simulink model "cx06_MA"  (Simulink 7.5)
settings: Solver=FixedStepDiscrete  StartTime=0.0  StopTime=10.0  RelTol=1e-3
undefined symbols (not defined in the file or in its folder): DiscIntNeverNeededParam, ECU555, int, motohawk_build_version, motohawk_trunc_name, motohawk_vardec_path
libraries: MotoHawk_lib x811, simulink x43, simulink_need_slupdate x1
(part 6 of 10)

== system cx06_MA/Inputs/Analog Inputs/Trans Inputs ==
  Bus Creator : BusCreator  Inputs=2
  Logical Operator : Logic  Operator=XOR  AllPortsSameDT=off  OutDataTypeMode=boolean  OutDataTypeStr=boolean
  Logical Operator1 : Logic  Operator=XOR  AllPortsSameDT=off  OutDataTypeMode=boolean  OutDataTypeStr=boolean
  motohawk_calibration : MotoHawk_lib/Calibration & Probing Blocks/motohawk_calibration  nam='Neutral_Invert'  val=1  storage=Calibration  show_more=on  name_source=Use Parameter  data_type=Inherit via back propagation  read_level=1  write_level=1  ovr_cals=on  view_as=Enumeration  enum_struct={'False', 'True'}  vector_style=Wide Row  use_help_units=off  help=''  units=''  use_header_enum=off  row_header_enum={}  col_header_enum={}  use_min_max=off  min_val=-inf  max_val=inf  use_precision=off  precision=''  gain=1  offset=0  exp=1  use_mototune_group=off  mototune_group=motohawk_vardec_path(gcb)
  motohawk_calibration1 : MotoHawk_lib/Calibration & Probing Blocks/motohawk_calibration  nam='Reverse_Invert'  val=0  storage=Calibration  show_more=on  name_source=Use Parameter  data_type=Inherit via back propagation  read_level=1  write_level=1  ovr_cals=on  view_as=Enumeration  enum_struct={'False', 'True'}  vector_style=Wide Row  use_help_units=off  help=''  units=''  use_header_enum=off  row_header_enum={}  col_header_enum={}  use_min_max=off  min_val=-inf  max_val=inf  use_precision=off  precision=''  gain=1  offset=0  exp=1  use_mototune_group=off  mototune_group=motohawk_vardec_path(gcb)
  motohawk_din : MotoHawk_lib/Digital I//O Blocks/motohawk_din  resource_name=[]  text_resource=DG1M  code_resource=RES_AN1M  val_resource=-1  target=ECU555-80  resource_enum_str=(None)=-1,AN1M=56,AN2M=57,AN3M=58,AN4M=59,AN5M=60,AN6M=61,AN7M=62,AN8M=63,AN9M=64,AN10M=65,AN11M=66,AN12M=67,AN13M=68,AN14M=69,AN15M=70,AN16M=71,AN17M=72,AN18M=73,AN19M=74,O2A=90,O2B=91,DG1M=93,DG2M=94,DG4M=96,ESTOP=97  pullup=None  use_stat=on  use_vardec=on  nam='Neutral'  read_level=1  write_level=1  group='I/O Pins | Inputs Config'
  motohawk_din1 : MotoHawk_lib/Digital I//O Blocks/motohawk_din  resource_name=[]  text_resource=AN3M  code_resource=RES_AN1M  val_resource=-1  target=ECU555-80  resource_enum_str=(None)=-1,AN1M=56,AN2M=57,AN3M=58,AN4M=59,AN5M=60,AN6M=61,AN7M=62,AN8M=63,AN9M=64,AN10M=65,AN11M=66,AN12M=67,AN13M=68,AN14M=69,AN15M=70,AN16M=71,AN17M=72,AN18M=73,AN19M=74,O2A=90,O2B=91,DG1M=93,DG2M=94,DG4M=96,ESTOP=97  pullup=None  use_stat=on  use_vardec=on  nam='Reverse'  read_level=1  write_level=1  group='I/O Pins | Inputs Config'
  motohawk_probe : MotoHawk_lib/Calibration & Probing Blocks/motohawk_probe  nam='cal_Neutral'  show_more=on  name_source=Use Parameter  read_level=1  view_as=Enumeration  enum_struct={'False', 'True'}  vector_style=Wide Row  use_help_units=off  help=''  units=''  use_header_enum=off  row_header_enum={}  col_header_enum={}  use_precision=off  precision=''  gain=1  offset=0  exp=1  use_mototune_group=off  mototune_group=motohawk_vardec_path(gcb)
  motohawk_probe1 : MotoHawk_lib/Calibration & Probing Blocks/motohawk_probe  nam='cal_Reverse'  show_more=on  name_source=Use Parameter  read_level=1  view_as=Enumeration  enum_struct={'False', 'True'}  vector_style=Wide Row  use_help_units=off  help=''  units=''  use_header_enum=off  row_header_enum={}  col_header_enum={}  use_precision=off  precision=''  gain=1  offset=0  exp=1  use_mototune_group=off  mototune_group=motohawk_vardec_path(gcb)
  motohawk_probe2 : MotoHawk_lib/Calibration & Probing Blocks/motohawk_probe  nam='Err_Reverse'  show_more=on  name_source=Use Parameter  read_level=1  view_as=Number  enum_struct={'Disabled', 'Enabled'}  vector_style=Wide Row  use_help_units=off  help=''  units=''  use_header_enum=off  row_header_enum={}  col_header_enum={}  use_precision=off  precision=''  gain=1  offset=0  exp=1  use_mototune_group=on  mototune_group='Debug | Inputs'
  motohawk_probe3 : MotoHawk_lib/Calibration & Probing Blocks/motohawk_probe  nam='Err_Neutral'  show_more=on  name_source=Use Parameter  read_level=1  view_as=Number  enum_struct={'Disabled', 'Enabled'}  vector_style=Wide Row  use_help_units=off  help=''  units=''  use_header_enum=off  row_header_enum={}  col_header_enum={}  use_precision=off  precision=''  gain=1  offset=0  exp=1  use_mototune_group=on  mototune_group='Debug | Inputs'
  Trans : Outport  OutDataType=sfix(16)  OutScaling=2^0
  wires:
  Bus Creator/1 -> Trans/1
  motohawk_calibration/1 -> Logical Operator/1
  motohawk_din/1 -> Logical Operator/2
  Logical Operator/1 -> Bus Creator/1, motohawk_probe/1  "Neutral"
  motohawk_calibration1/1 -> Logical Operator1/1
  motohawk_din1/1 -> Logical Operator1/2
  Logical Operator1/1 -> motohawk_probe1/1, Bus Creator/2  "Reverse"
  motohawk_din/2 -> motohawk_probe3/1
  motohawk_din1/2 -> motohawk_probe2/1

== system cx06_MA/Inputs/GMLAN Inputs/Valid_Chk ==
  In : Inport  OutDataType=sfix(16)  OutScaling=2^0
  Valid : Inport  Port=2  OutDataType=sfix(16)  OutScaling=2^0
  Switch : Switch  Criteria=u2 ~= 0
  Unit Delay : UnitDelay  SampleTime=-1
  Out1 : Outport  OutDataType=sfix(16)  OutScaling=2^0
  wires:
  Valid/1 -> Switch/2
  In/1 -> Switch/3
  Unit Delay/1 -> Switch/1
  Switch/1 -> Unit Delay/1, Out1/1

== system cx06_MA/Inputs/GMLAN Inputs/Valid_Chk1 ==
  In : Inport  OutDataType=sfix(16)  OutScaling=2^0
  Valid : Inport  Port=2  OutDataType=sfix(16)  OutScaling=2^0
  Switch : Switch  Criteria=u2 ~= 0
  Unit Delay : UnitDelay  SampleTime=-1
  Out1 : Outport  OutDataType=sfix(16)  OutScaling=2^0
  wires:
  Switch/1 -> Out1/1, Unit Delay/1
  Unit Delay/1 -> Switch/1
  In/1 -> Switch/3
  Valid/1 -> Switch/2

== system cx06_MA/Inputs/GMLAN Inputs/Valid_Chk2 ==
  In : Inport  OutDataType=sfix(16)  OutScaling=2^0
  Valid : Inport  Port=2  OutDataType=sfix(16)  OutScaling=2^0
  Switch : Switch  Criteria=u2 ~= 0
  Unit Delay : UnitDelay  SampleTime=-1
  Out1 : Outport  OutDataType=sfix(16)  OutScaling=2^0
  wires:
  Valid/1 -> Switch/2
  In/1 -> Switch/3
  Unit Delay/1 -> Switch/1
  Switch/1 -> Unit Delay/1, Out1/1

== system cx06_MA/Inputs/GMLAN Inputs/Valid_Chk3 ==
  In : Inport  OutDataType=sfix(16)  OutScaling=2^0
  Valid : Inport  Port=2  OutDataType=sfix(16)  OutScaling=2^0
  Switch : Switch  Criteria=u2 ~= 0
  Unit Delay : UnitDelay  SampleTime=-1
  Out1 : Outport  OutDataType=sfix(16)  OutScaling=2^0
  wires:
  Switch/1 -> Out1/1, Unit Delay/1
  Unit Delay/1 -> Switch/1
  In/1 -> Switch/3
  Valid/1 -> Switch/2

== system cx06_MA/Inputs/IPT CAN Input/speed_calc ==
  whl_rpm : Inport  OutDataType=sfix(16)  OutScaling=2^0
  gear_ratio : Inport  Port=2  OutDataType=sfix(16)  OutScaling=2^0
  Constant : Constant  Value=pi()/12/5280*60  OutDataType=sfix(16)  OutScaling=2^0
  Divide : Product  Inputs=***/  OutDataType=sfix(16)  OutScaling=2^-10
  motohawk_calibration : MotoHawk_lib/Calibration & Probing Blocks/motohawk_calibration  nam='Tire_Size'  val=26  storage=Calibration  show_more=on  name_source=Use Parameter  data_type=Inherit from 'Default Value'  read_level=1  write_level=1  ovr_cals=on  view_as=Number  enum_struct={'Disabled', 'Enabled'}  vector_style=Wide Row  use_help_units=on  help='Tire Diameter (used to calculate vehicle speed'  units='in'  use_header_enum=off  row_header_enum={}  col_header_enum={}  use_min_max=off  min_val=0  max_val=100  use_precision=on  precision='2.2'  gain=1  offset=0  exp=1  use_mototune_group=off  mototune_group=motohawk_vardec_path(gcb)
  Veh_mph : Outport  OutDataType=sfix(16)  OutScaling=2^0
  wires:
  whl_rpm/1 -> Divide/1
  Constant/1 -> Divide/2
  motohawk_calibration/1 -> Divide/3
  Divide/1 -> Veh_mph/1
  gear_ratio/1 -> Divide/4

== system cx06_MA/Outputs/Analog Outputs/Backup_Relay_Control ==
  Engine_Start_In : Inport  OutDataType=sfix(16)  OutScaling=2^0
  Chart : Stateflow chart  TreatAsAtomicUnit=on
  Data Type Conversion : DataTypeConversion  OutDataTypeMode=boolean  OutDataType=sfix(16)  OutScaling=2^0  OutDataTypeStr=boolean
  Data Type Conversion1 : DataTypeConversion  OutDataTypeMode=boolean  OutDataType=sfix(16)  OutScaling=2^0  OutDataTypeStr=boolean
  Subsystem : Subsystem
  Unit Delay : UnitDelay  SampleTime=-1
  motohawk_calibration : MotoHawk_lib/Calibration & Probing Blocks/motohawk_calibration  nam='Idle_to_Crank_Delay'  val=5  storage=Calibration  show_more=on  name_source=Use Parameter  data_type=uint16  read_level=1  write_level=1  ovr_cals=on  view_as=Number  enum_struct={'Disabled', 'Enabled'}  vector_style=Wide Row  use_help_units=on  help=''  units='ms'  use_header_enum=off  row_header_enum={}  col_header_enum={}  use_min_max=on  min_val=0  max_val=1000  use_precision=on  precision=''  gain=1/5  offset=0  exp=1  use_mototune_group=off  mototune_group=motohawk_vardec_path(gcb)
  motohawk_calibration1 : MotoHawk_lib/Calibration & Probing Blocks/motohawk_calibration  nam='Crank_to_Idle_Delay'  val=5  storage=Calibration  show_more=on  name_source=Use Parameter  data_type=uint16  read_level=1  write_level=1  ovr_cals=on  view_as=Number  enum_struct={'Disabled', 'Enabled'}  vector_style=Wide Row  use_help_units=on  help=''  units='ms'  use_header_enum=off  row_header_enum={}  col_header_enum={}  use_min_max=on  min_val=0  max_val=1000  use_precision=on  precision=''  gain=1/5  offset=0  exp=1  use_mototune_group=off  mototune_group=motohawk_vardec_path(gcb)
  motohawk_probe : MotoHawk_lib/Calibration & Probing Blocks/motohawk_probe  nam='KevOBox_State'  show_more=on  name_source=Use Parameter  read_level=1  view_as=Enumeration  enum_struct={'Idle', 'About_to_Crank', 'Crank', 'About_to_Idle'}  vector_style=Wide Row  use_help_units=off  help=''  units=''  use_header_enum=off  row_header_enum={}  col_header_enum={}  use_precision=off  precision=''  gain=1  offset=0  exp=1  use_mototune_group=off  mototune_group=motohawk_vardec_path(gcb)
  motohawk_probe1 : MotoHawk_lib/Calibration & Probing Blocks/motohawk_probe  nam='Timer'  show_more=on  name_source=Use Parameter  read_level=1  view_as=Number  enum_struct={'Idle', 'About_to_Crank',Crank',About_to_Idle'}  vector_style=Wide Row  use_help_units=off  help=''  units=''  use_header_enum=off  row_header_enum={}  col_header_enum={}  use_precision=off  precision=''  gain=1  offset=0  exp=1  use_mototune_group=off  mototune_group=motohawk_vardec_path(gcb)
  Engine_Start_Out : Outport  OutDataType=sfix(16)  OutScaling=2^0
  Clarion_Pwr_Out : Outport  Port=2  OutDataType=sfix(16)  OutScaling=2^0
  wires:
  motohawk_calibration/1 -> Subsystem/2(Idle_to_Crank Cal)
  motohawk_calibration1/1 -> Subsystem/3(Crank_to_Idle Cal)
  Chart/4(state) -> motohawk_probe/1
  Chart/3(timer) -> Unit Delay/1
  Chart/1(LSD_Eng) -> Data Type Conversion/1
  Chart/2(LSD_Nav) -> Data Type Conversion1/1
  Subsystem/2(Idle_to_Crank Delay) -> Chart/2(Delay_1)
  Subsystem/3(Crank_to_Idle Delay) -> Chart/3(Delay_2)
  Subsystem/1(Timer) -> motohawk_probe1/1
  Engine_Start_In/1 -> Chart/1(Eng_Start)
  Data Type Conversion1/1 -> Clarion_Pwr_Out/1
  Data Type Conversion/1 -> Engine_Start_Out/1
  Unit Delay/1 -> Subsystem/1(timer_en)

== system cx06_MA/Outputs/Analog Outputs/Nav Sys Timer ==
  Constant1 : Constant  OutDataType=sfix(16)  OutScaling=2^0
  Gain1 : Gain  Gain=1/200  ParameterDataType=sfix(16)  ParameterScaling=2^0  OutDataType=sfix(16)  OutScaling=2^0
  Relational Operator1 : RelationalOperator  Operator=>  LogicOutDataTypeMode=Specify via dialog  OutDataTypeStr=uint(8)
  Saturation : Saturate  UpperLimit=6000  LowerLimit=0
  Sum : Sum  Inputs=|++  OutDataType=sfix(16)  OutScaling=2^0
  Unit Delay : UnitDelay  X0=1  SampleTime=-1
  motohawk_calibration2 : MotoHawk_lib/Calibration & Probing Blocks/motohawk_calibration  nam='Disable_Nav_Safety_Delay'  val=3000  storage=Calibration  show_more=on  name_source=Use Parameter  data_type=double  read_level=1  write_level=1  ovr_cals=on  view_as=Number  enum_struct={'False', 'True'}  vector_style=Wide Row  use_help_units=on  help='time which requested IPT Torque has to be below Zero_Threshold before disabling MCU'  units='sec'  use_header_enum=off  row_header_enum={}  col_header_enum={}  use_min_max=on  min_val=0  max_val=6000  use_precision=on  precision='1.3'  gain=1/200  offset=0  exp=1  use_mototune_group=off  mototune_group=motohawk_vardec_path(gcb)
  motohawk_probe1 : MotoHawk_lib/Calibration & Probing Blocks/motohawk_probe  nam='Nav_Cnt_Seconds'  show_more=off  name_source=Use Parameter  read_level=1  view_as=Number  enum_struct={'Disabled', 'Enabled'}  vector_style=Wide Row  use_help_units=off  help=''  units=''  use_header_enum=off  row_header_enum={}  col_header_enum={}  use_precision=off  precision=''  gain=1  offset=0  exp=1  use_mototune_group=off  mototune_group=motohawk_vardec_path(gcb)
  Out : Outport  OutDataType=sfix(16)  OutScaling=2^0
  wires:
  motohawk_calibration2/1 -> Relational Operator1/2
  Relational Operator1/1 -> Out/1
  Sum/1 -> Saturation/1
  Saturation/1 -> Unit Delay/1, Relational Operator1/1, Gain1/1
  Unit Delay/1 -> Sum/1
  Constant1/1 -> Sum/2
  Gain1/1 -> motohawk_probe1/1

== system cx06_MA/Outputs/Drive-by-Wire CAN Output/Subsystem ==
  Reset_AO1 : Inport  OutDataType=sfix(16)  OutScaling=2^0
  Output1 : Inport  Port=2  OutDataType=sfix(16)  OutScaling=2^0
  Reset_AO2 : Inport  Port=3  OutDataType=sfix(16)  OutScaling=2^0
  Output2 : Inport  Port=4  OutDataType=sfix(16)  OutScaling=2^0
  Bitwise Operator : simulink/Logic and Bit Operations/Bitwise Operator  logicop=AND  UseBitMask=on  BitMask=1  BitMaskRealWorld=Stored Integer
  Bitwise Operator1 : simulink/Logic and Bit Operations/Bitwise Operator  logicop=AND  UseBitMask=on  BitMask=1  BitMaskRealWorld=Stored Integer
  Bitwise Operator2 : simulink/Logic and Bit Operations/Bitwise Operator  logicop=AND  UseBitMask=on  BitMask=hex2dec('FFF')  BitMaskRealWorld=Stored Integer
  Bitwise Operator3 : simulink/Logic and Bit Operations/Bitwise Operator  logicop=OR  UseBitMask=off  NumInputPorts=2  BitMask=hex2dec('FFF')  BitMaskRealWorld=Stored Integer
  Bitwise Operator4 : simulink/Logic and Bit Operations/Bitwise Operator  logicop=AND  UseBitMask=on  BitMask=hex2dec('FFF')  BitMaskRealWorld=Stored Integer
  Bitwise Operator5 : simulink/Logic and Bit Operations/Bitwise Operator  logicop=OR  UseBitMask=off  NumInputPorts=2  BitMask=hex2dec('FFF')  BitMaskRealWorld=Stored Integer
  Bitwise Operator6 : simulink/Logic and Bit Operations/Bitwise Operator  logicop=XOR  UseBitMask=off  NumInputPorts=4  BitMask=hex2dec('FFF')  BitMaskRealWorld=Stored Integer
  Extract Bits : simulink/Logic and Bit Operations/Extract Bits  SystemSampleTime=-1  bitsToExtract=Range starting with most significant bit  numBits=8  bitIdxRange=[0 7]  outScalingMode=Treat bit field as an integer
  Extract Bits1 : simulink/Logic and Bit Operations/Extract Bits  SystemSampleTime=-1  bitsToExtract=Range ending with least significant bit  numBits=8  bitIdxRange=[0 7]  outScalingMode=Treat bit field as an integer
  Extract Bits2 : simulink/Logic and Bit Operations/Extract Bits  SystemSampleTime=-1  bitsToExtract=Range starting with most significant bit  numBits=8  bitIdxRange=[0 7]  outScalingMode=Treat bit field as an integer
  Extract Bits3 : simulink/Logic and Bit Operations/Extract Bits  SystemSampleTime=-1  bitsToExtract=Range ending with least significant bit  numBits=8  bitIdxRange=[0 7]  outScalingMode=Treat bit field as an integer
  Shift Arithmetic : simulink/Logic and Bit Operations/Shift Arithmetic  SystemSampleTime=-1  nBitShiftRight=-4  nBinPtShiftRight=0
  Checksum : Outport  OutDataType=sfix(16)  OutScaling=2^0
  wires:
  Reset_AO1/1 -> Bitwise Operator/1
  Bitwise Operator/1 -> Shift Arithmetic/1
  Reset_AO2/1 -> Bitwise Operator1/1
  Shift Arithmetic/1 -> Bitwise Operator3/1
  Bitwise Operator2/1 -> Bitwise Operator3/2
  Bitwise Operator4/1 -> Bitwise Operator5/2
  Output2/1 -> Bitwise Operator4/1
  Bitwise Operator1/1 -> Bitwise Operator5/1
  Bitwise Operator3/1 -> Extract Bits/1, Extract Bits1/1
  Bitwise Operator5/1 -> Extract Bits2/1, Extract Bits3/1
  Extract Bits/1 -> Bitwise Operator6/1
  Extract Bits1/1 -> Bitwise Operator6/2
  Extract Bits2/1 -> Bitwise Operator6/3
  Extract Bits3/1 -> Bitwise Operator6/4
  Bitwise Operator6/1 -> Checksum/1
  Output1/1 -> Bitwise Operator2/1

== system cx06_MA/Outputs/GMLAN Outputs/Fuel/SOC_Gage_Conditioning ==
  In1 : Inport  OutDataType=sfix(16)  OutScaling=2^0
  Bus Selector2 : BusSelector  OutputSignals=Analog.Fuel_Level,Analog.cruiseBut,JCI.SOC
  Constant : Constant  Value=0  OutDataType=sfix(16)  OutScaling=2^0
  Constant1 : Constant  OutDataType=fixdt(1, 16)  OutScaling=2^0
  Constant2 : Constant  Value=0  OutDataType=sfix(16)  OutScaling=2^0
  Constant3 : Constant  OutDataType=sfix(16)  OutScaling=2^0
  Fuel_Signal_Conditioning : Subsystem
  Gain : Gain  Gain=100  ParameterDataType=sfix(16)  ParameterScaling=2^0  OutDataType=sfix(16)  OutScaling=2^0
  Logical Operator : Logic  Operator=NOT  AllPortsSameDT=off  OutDataTypeMode=Specify via dialog  OutDataTypeStr=uint(8)
  Mux4 : Mux  Inputs=3
  Relational Operator : RelationalOperator  Operator===  LogicOutDataTypeMode=boolean  OutDataTypeStr=boolean
  Relational Operator1 : RelationalOperator  Operator===  LogicOutDataTypeMode=boolean  OutDataTypeStr=boolean
  Relational Operator2 : RelationalOperator  Operator===  LogicOutDataTypeMode=boolean  OutDataTypeStr=boolean
  Saturation : Saturate  UpperLimit=1000  LowerLimit=0
  Saturation1 : Saturate  UpperLimit=100  LowerLimit=0
  Saturation3 : Saturate  UpperLimit=100  LowerLimit=0
  Sum : Sum  Inputs=-+  OutDataType=sfix(16)  OutScaling=2^0
  Sum1 : Sum  Inputs=|++  OutDataType=sfix(16)  OutScaling=2^0
  Switch{,1..3} (4 alike) : Switch  Threshold=1
  Unit Delay : UnitDelay  X0=1  SampleTime=-1
  Unit Delay1 : UnitDelay  X0=1001  SampleTime=-1
  motohawk_calibration : MotoHawk_lib/Calibration & Probing Blocks/motohawk_calibration  nam='Gage_Delay'  val=0  storage=Calibration  show_more=on  name_source=Use Parameter  data_type=Inherit from 'Default Value'  read_level=1  write_level=1  ovr_cals=on  view_as=Number  enum_struct={'Disabled', 'Enabled'}  vector_style=Wide Row  use_help_units=off  help=''  units=''  use_header_enum=off  row_header_enum={}  col_header_enum={}  use_min_max=on  min_val=0  max_val=5  use_precision=on  precision='1.3'  gain=1/200  offset=0  exp=1  use_mototune_group=off  mototune_group=motohawk_vardec_path(gcb)
  motohawk_calibration1 : MotoHawk_lib/Calibration & Probing Blocks/motohawk_calibration  nam='TransGoToPoint'  val=12  storage=Calibration  show_more=on  name_source=Use Parameter  data_type=Inherit from 'Default Value'  read_level=1  write_level=1  ovr_cals=on  view_as=Number  enum_struct={'Disabled', 'Enabled'}  vector_style=Wide Row  use_help_units=off  help=''  units=''  use_header_enum=off  row_header_enum={}  col_header_enum={}  use_min_max=on  min_val=0  max_val=100  use_precision=on  precision='1.3'  gain=1  offset=0  exp=1  use_mototune_group=off  mototune_group=motohawk_vardec_path(gcb)
  motohawk_calibration2 : MotoHawk_lib/Calibration & Probing Blocks/motohawk_calibration  nam='Bat_Lvl_Offset'  val=0  storage=Calibration  show_more=on  name_source=Use Parameter  data_type=Inherit from 'Default Value'  read_level=1  write_level=1  ovr_cals=on  view_as=Number  enum_struct={'Disabled', 'Enabled'}  vector_style=Wide Row  use_help_units=off  help=''  units=''  use_header_enum=off  row_header_enum={}  col_header_enum={}  use_min_max=on  min_val=0  max_val=100  use_precision=on  precision='1.3'  gain=1  offset=0  exp=1  use_mototune_group=off  mototune_group=motohawk_vardec_path(gcb)
  motohawk_calibration7 : MotoHawk_lib/Calibration & Probing Blocks/motohawk_calibration  nam='SOC_Lvl_Zero'  val=5  storage=Calibration  show_more=on  name_source=Use Parameter  data_type=Inherit via back propagation  read_level=1  write_level=1  ovr_cals=on  view_as=Number  enum_struct={'Disabled', 'Enabled'}  vector_style=Wide Row  use_help_units=off  help=''  units=''  use_header_enum=off  row_header_enum={}  col_header_enum={}  use_min_max=off  min_val=-inf  max_val=inf  use_precision=off  precision=''  gain=1  offset=0  exp=1  use_mototune_group=off  mototune_group=motohawk_vardec_path(gcb)
  motohawk_calibration8 : MotoHawk_lib/Calibration & Probing Blocks/motohawk_calibration  nam='SOC_Lvl_Full'  val=100  storage=Calibration  show_more=on  name_source=Use Parameter  data_type=Inherit via back propagation  read_level=1  write_level=1  ovr_cals=on  view_as=Number  enum_struct={'Disabled', 'Enabled'}  vector_style=Wide Row  use_help_units=off  help=''  units=''  use_header_enum=off  row_header_enum={}  col_header_enum={}  use_min_max=off  min_val=-inf  max_val=inf  use_precision=off  precision=''  gain=1  offset=0  exp=1  use_mototune_group=off  mototune_group=motohawk_vardec_path(gcb)
  motohawk_probe : MotoHawk_lib/Calibration & Probing Blocks/motohawk_probe  nam='Bat_Lvl_Out'  show_more=off  name_source=Use Parameter  read_level=1  view_as=Number  enum_struct={'Disabled', 'Enabled'}  vector_style=Wide Row  use_help_units=off  help=''  units=''  use_header_enum=off  row_header_enum={}  col_header_enum={}  use_precision=off  precision=''  gain=1  offset=0  exp=1  use_mototune_group=off  mototune_group=motohawk_vardec_path(gcb)
  motohawk_probe1 : MotoHawk_lib/Calibration & Probing Blocks/motohawk_probe  nam='Fuel_Lvl_Out'  show_more=off  name_source=Use Parameter  read_level=1  view_as=Number  enum_struct={'Disabled', 'Enabled'}  vector_style=Wide Row  use_help_units=off  help=''  units=''  use_header_enum=off  row_header_enum={}  col_header_enum={}  use_precision=off  precision=''  gain=1  offset=0  exp=1  use_mototune_group=off  mototune_group=motohawk_vardec_path(gcb)
  motohawk_probe2 : MotoHawk_lib/Calibration & Probing Blocks/motohawk_probe  nam='Delay_Count'  show_more=off  name_source=Use Parameter  read_level=1  view_as=Number  enum_struct={'Disabled', 'Enabled'}  vector_style=Wide Row  use_help_units=off  help=''  units=''  use_header_enum=off  row_header_enum={}  col_header_enum={}  use_precision=off  precision=''  gain=1  offset=0  exp=1  use_mototune_group=off  mototune_group=motohawk_vardec_path(gcb)
  my2pt Cal : Fcn  Expr=(u[1]-u[3])/(u[2]-u[3])
  Out1 : Outport  OutDataType=sfix(16)  OutScaling=2^0
  wires:
  In1/1 -> Bus Selector2/1
  Bus Selector2/1 -> Fuel_Signal_Conditioning/1(Fuel_Level)  "<Fuel_Level>"
  Bus Selector2/2 -> Relational Operator/1  "<cruiseBut>"
  Constant/1 -> Relational Operator/2, Switch3/1
  Relational Operator/1 -> Switch/2, Unit Delay/1, Relational Operator1/1
  Fuel_Signal_Conditioning/1(Out1) -> Switch/1, motohawk_probe1/1
  Switch/1 -> Switch1/1
  Unit Delay/1 -> Relational Operator1/2
  Constant2/1 -> Relational Operator2/1
  Relational Operator2/1 -> Switch1/2
  Saturation/1 -> Relational Operator2/2, Unit Delay1/1, motohawk_probe2/1
  Sum/1 -> Saturation/1
  Constant3/1 -> Sum/1
  Relational Operator1/1 -> Switch2/2
  Unit Delay1/1 -> Switch2/1
  motohawk_calibration/1 -> Switch2/3
  Switch2/1 -> Sum/2
  Mux4/1 -> my2pt Cal/1
  motohawk_calibration7/1 -> Mux4/3
  motohawk_calibration8/1 -> Mux4/2
  Bus Selector2/3 -> Mux4/1  "<SOC>"
  motohawk_calibration1/1 -> Switch1/3
  Switch1/1 -> Out1/1
  motohawk_calibration2/1 -> Sum1/2
  Switch3/1 -> Switch/3
  Saturation3/1 -> Switch3/3
  Logical Operator/1 -> Switch3/2
  my2pt Cal/1 -> Gain/1
  Gain/1 -> Saturation1/1
  Sum1/1 -> Saturation3/1, motohawk_probe/1
  Saturation1/1 -> Sum1/1
  Constant1/1 -> Logical Operator/1

== system cx06_MA/Outputs/GMLAN Outputs/Speed_Integrator ==
  In1 : Inport  OutDataType=sfix(16)  OutScaling=2^0
  Compare To Constant : simulink/Logic and Bit Operations/Compare To Constant  SystemSampleTime=-1  relop=>  const=1000  LogicOutDataTypeMode=uint8  ZeroCross=off
  Compare To Constant1 : simulink/Logic and Bit Operations/Compare To Constant  SystemSampleTime=-1  relop=<  const=5  LogicOutDataTypeMode=uint8  ZeroCross=off
  Gain : Gain  Gain=1/(60*60*200)  ParameterDataType=sfix(16)  ParameterScaling=2^0  OutDataType=sfix(16)  OutScaling=2^0
  Logical Operator : Logic  Operator=NOT  AllPortsSameDT=off  OutDataTypeMode=Specify via dialog  OutDataTypeStr=uint(8)
  Logical Operator1 : Logic  Operator=OR  AllPortsSameDT=off  OutDataTypeMode=Specify via dialog  OutDataTypeStr=uint(8)
  Product : Product  OutDataType=sfix(16)  OutScaling=2^0  RndMeth=Zero
  Sum : Sum  Inputs=|++  OutDataType=sfix(16)  OutScaling=2^0
  Unit Delay : UnitDelay  SampleTime=-1
  Reset : Outport  OutDataType=sfix(16)  OutScaling=2^0
  Out1 : Outport  Port=2  OutDataType=sfix(16)  OutScaling=2^0
  wires:
  In1/1 -> Gain/1
  Gain/1 -> Sum/1
  Unit Delay/1 -> Sum/2
  Sum/1 -> Compare To Constant/1, Product/1, Out1/1, Compare To Constant1/1
  Compare To Constant/1 -> Logical Operator/1, Logical Operator1/2
  Product/1 -> Unit Delay/1
  Logical Operator/1 -> Product/2
  Logical Operator1/1 -> Reset/1
  Compare To Constant1/1 -> Logical Operator1/1

== system cx06_MA/Outputs/GMLAN Outputs/Subsystem ==
  Engine_Running : Inport  OutDataType=sfix(16)  OutScaling=2^0
  Constant : Constant  OutDataType=sfix(16)  OutScaling=2^0
  Switch : Switch  Criteria=u2 ~= 0
  motohawk_fault_action : MotoHawk_lib/Fault Management Blocks/motohawk_fault_action  nam='Clutch'  output_status=on  eval_nam=Clutch
  Out1 : Outport  OutDataType=sfix(16)  OutScaling=2^0
  wires:
  motohawk_fault_action/1 -> Switch/2
  Constant/1 -> Switch/3
  Engine_Running/1 -> Switch/1
  Switch/1 -> Out1/1

== system cx06_MA/Outputs/IPT CAN Output/MCU_Management ==
  Motor_Torque_Request : Inport  OutDataType=sfix(16)  OutScaling=2^0
  MCU_Enable_IN : Inport  Port=2  OutDataType=sfix(16)  OutScaling=2^0
  Abs : Abs
  Constant : Constant  Value=0  OutDataType=sfix(16)  OutScaling=2^0
  Constant1 : Constant  OutDataType=sfix(16)  OutScaling=2^0
  Data Type Conversion : DataTypeConversion  OutDataTypeMode=uint8  OutDataType=sfix(16)  OutScaling=2^0  OutDataTypeStr=uint8
  Gain1 : Gain  Gain=1/200  ParameterDataType=sfix(16)  ParameterScaling=2^0  OutDataType=sfix(16)  OutScaling=2^0
  Logical Operator : Logic  Operator=OR  AllPortsSameDT=off  OutDataTypeMode=boolean  OutDataTypeStr=boolean
  Relational Operator : RelationalOperator  Operator=<  LogicOutDataTypeMode=Specify via dialog  OutDataTypeStr=uint(8)
  Relational Operator1 : RelationalOperator  Operator=<  LogicOutDataTypeMode=Specify via dialog  OutDataTypeStr=uint(8)
  Saturation : Saturate  UpperLimit=6000  LowerLimit=0
  Sum : Sum  Inputs=|++  OutDataType=sfix(16)  OutScaling=2^0
  Switch : Switch  Criteria=u2 > Threshold  OutDataTypeStr=Inherit: Inherit via back propagation  RndMeth=Nearest
  Switch1 : Switch  Criteria=u2 > Threshold  OutDataTypeStr=Inherit: Inherit via back propagation
  Unit Delay : UnitDelay  X0=1  SampleTime=-1
  motohawk_calibration1 : MotoHawk_lib/Calibration & Probing Blocks/motohawk_calibration  nam='MCU_Manage_Source'  val=0  storage=Calibration  show_more=on  name_source=Use Parameter  data_type=uint8  read_level=1  write_level=1  ovr_cals=on  view_as=Enumeration  enum_struct={'By_State', 'By_Torque_Dmd'}  vector_style=Wide Row  use_help_units=off  help=''  units=''  use_header_enum=off  row_header_enum={}  col_header_enum={}  use_min_max=on  min_val=0  max_val=1  use_precision=off  precision=''  gain=1  offset=0  exp=1  use_mototune_group=off  mototune_group=motohawk_vardec_path(gcb)
  motohawk_calibration11 : MotoHawk_lib/Calibration & Probing Blocks/motohawk_calibration  nam='Zero_Threshold'  val=.01  storage=Calibration  show_more=on  name_source=Use Parameter  data_type=double  read_level=1  write_level=1  ovr_cals=on  view_as=Number  enum_struct={'False', 'True'}  vector_style=Wide Row  use_help_units=off  help=''  units=''  use_header_enum=off  row_header_enum={}  col_header_enum={}  use_min_max=on  min_val=0  max_val=1  use_precision=on  precision='1.3'  gain=1  offset=0  exp=1  use_mototune_group=off  mototune_group=motohawk_vardec_path(gcb)
  motohawk_calibration2 : MotoHawk_lib/Calibration & Probing Blocks/motohawk_calibration  nam='Disable_MCU_Delay'  val=1200  storage=Calibration  show_more=on  name_source=Use Parameter  data_type=double  read_level=1  write_level=1  ovr_cals=on  view_as=Number  enum_struct={'False', 'True'}  vector_style=Wide Row  use_help_units=on  help='time which requested IPT Torque has to be below Zero_Threshold before disabling MCU'  units='sec'  use_header_enum=off  row_header_enum={}  col_header_enum={}  use_min_max=on  min_val=0  max_val=6000  use_precision=on  precision='1.3'  gain=1/200  offset=0  exp=1  use_mototune_group=off  mototune_group=motohawk_vardec_path(gcb)
  motohawk_calibration3 : MotoHawk_lib/Calibration & Probing Blocks/motohawk_calibration  nam='Inhibit_MCU_Management'  val=1  storage=Calibration  show_more=on  name_source=Use Parameter  data_type=uint8  read_level=1  write_level=1  ovr_cals=on  view_as=Enumeration  enum_struct={'False', 'True'}  vector_style=Wide Row  use_help_units=off  help=''  units=''  use_header_enum=off  row_header_enum={}  col_header_enum={}  use_min_max=on  min_val=0  max_val=1  use_precision=off  precision=''  gain=1  offset=0  exp=1  use_mototune_group=off  mototune_group=motohawk_vardec_path(gcb)
  motohawk_probe : MotoHawk_lib/Calibration & Probing Blocks/motohawk_probe  nam='Below_Thres_Comparison'  show_more=off  name_source=Use Parameter  read_level=1  view_as=Number  enum_struct={'Disabled', 'Enabled'}  vector_style=Wide Row  use_help_units=off  help=''  units=''  use_header_enum=off  row_header_enum={}  col_header_enum={}  use_precision=off  precision=''  gain=1  offset=0  exp=1  use_mototune_group=off  mototune_group=motohawk_vardec_path(gcb)
  motohawk_probe1 : MotoHawk_lib/Calibration & Probing Blocks/motohawk_probe  nam='Cnt_Seconds'  show_more=off  name_source=Use Parameter  read_level=1  view_as=Number  enum_struct={'Disabled', 'Enabled'}  vector_style=Wide Row  use_help_units=off  help=''  units=''  use_header_enum=off  row_header_enum={}  col_header_enum={}  use_precision=off  precision=''  gain=1  offset=0  exp=1  use_mototune_group=off  mototune_group=motohawk_vardec_path(gcb)
  MCU_Enable_OUT : Outport  OutDataType=sfix(16)  OutScaling=2^0
  wires:
  motohawk_calibration1/1 -> Switch/2
  MCU_Enable_IN/1 -> Switch/3
  Motor_Torque_Request/1 -> Abs/1
  Abs/1 -> Relational Operator/1
  motohawk_calibration11/1 -> Relational Operator/2
  Relational Operator/1 -> Data Type Conversion/1
  Data Type Conversion/1 -> Switch1/2, motohawk_probe/1
  motohawk_calibration2/1 -> Relational Operator1/2
  Relational Operator1/1 -> Switch/1
  Switch1/1 -> Saturation/1
  Saturation/1 -> Unit Delay/1, Relational Operator1/1, Gain1/1
  Constant/1 -> Switch1/3
  Unit Delay/1 -> Sum/1
  Constant1/1 -> Sum/2
  Sum/1 -> Switch1/1
  Gain1/1 -> motohawk_probe1/1
  Switch/1 -> Logical Operator/1
  motohawk_calibration3/1 -> Logical Operator/2
  Logical Operator/1 -> MCU_Enable_OUT/1

== system cx06_MA/Strategy/Fiat/GMLAN Control Code/Gear Calc ==
  In1 : Inport  OutDataType=sfix(16)  OutScaling=2^0
  gear_In : Inport  Port=2  OutDataType=sfix(16)  OutScaling=2^0
  Bus Selector : BusSelector  OutputSignals=Analog.Driver.Clutch,Analog.Trans.Neutral,Analog.Trans.Reverse
  Constant : Constant  Value=-1  OutDataTypeMode=int8  OutDataType=sfix(16)  OutScaling=2^0  OutDataTypeStr=int8
  Logical Operator : Logic  Operator=OR  AllPortsSameDT=off  OutDataTypeMode=boolean  OutDataTypeStr=boolean
  Logical Operator1 : Logic  Operator=NOT  AllPortsSameDT=off  OutDataTypeMode=boolean  OutDataTypeStr=boolean
  Product : Product  OutDataTypeMode=int8  OutDataType=sfix(16)  OutScaling=2^0  OutDataTypeStr=int8  RndMeth=Zero
  Relational Operator : RelationalOperator  Operator=<=  LogicOutDataTypeMode=boolean  OutDataTypeStr=boolean
  Switch : Switch  Criteria=u2 ~= 0
  motohawk_data_read : MotoHawk_lib/Data Storage Blocks/motohawk_data_read  source=Lookup By Name  structure=Scalar  operation=Read scalar from location by index  sz_vec=4  sz_row=2  sz_col=3  typ=double  nam='AT_Stop'  checkNull=on  struct_inst_name='Struct1'  struct_nam='MyStruct'
  motohawk_probe : MotoHawk_lib/Calibration & Probing Blocks/motohawk_probe  nam='Gear'  show_more=on  name_source=Use Parameter  read_level=1  view_as=Number  enum_struct={'Disabled', 'Enabled'}  vector_style=Wide Row  use_help_units=off  help=''  units=''  use_header_enum=off  row_header_enum={}  col_header_enum={}  use_precision=off  precision=''  gain=1  offset=0  exp=1  use_mototune_group=off  mototune_group=motohawk_vardec_path(gcb)
  gear : Outport  OutDataType=sfix(16)  OutScaling=2^0
  wires:
  In1/1 -> Bus Selector/1
  Product/1 -> gear/1, motohawk_probe/1
  Bus Selector/3 -> Switch/2  "<Reverse>"
  Constant/1 -> Switch/1
  motohawk_data_read/1 -> Relational Operator/1
  Bus Selector/1 -> Relational Operator/2  "<Clutch>"
  Relational Operator/1 -> Logical Operator/1
  Bus Selector/2 -> Logical Operator/2  "<Neutral>"
  Logical Operator/1 -> Logical Operator1/1
  Logical Operator1/1 -> Product/1
  Switch/1 -> Product/2
  gear_In/1 -> Switch/3

== system cx06_MA/Strategy/Fiat/GMLAN Control Code/Gear_Estimation ==
  In1 : Inport  OutDataType=sfix(16)  OutScaling=2^0
  Abs : Abs
  Add : Sum  OutDataType=sfix(16)  OutScaling=2^-10  InputSameDT=on  OutDataTypeStr=Inherit: Same as first input
  Add1 : Sum  Inputs=++++++  OutDataTypeMode=int8  OutDataType=sfix(16)  OutScaling=2^-10  OutDataTypeStr=int8
  Bus Selector1 : BusSelector  OutputSignals=GMLAN.FL_Whl_Spd,GMLAN.FR_Whl_Spd,Fiat.Engine Speed and Pedal Pos.Eng_Spd
  Compare To Zero1 : simulink/Logic and Bit Operations/Compare To Zero  SystemSampleTime=-1  relop===  LogicOutDataTypeMode=uint8  ZeroCross=off
  Demux : Demux  Outputs=6
  Divide : Product  Inputs=**  OutDataType=sfix(16)  OutScaling=2^-10
  Divide1 : Product  Inputs=**  OutDataType=sfix(16)  OutScaling=2^-10
  Gain : Gain  Gain=0.5  ParameterDataType=sfix(16)  ParameterScaling=2^0  OutDataType=sfix(16)  OutScaling=2^0  OutDataTypeStr=Inherit: Same as input
  Gain1 : Gain  ParameterDataType=sfix(16)  ParameterScaling=2^0  OutDataType=sfix(16)  OutScaling=2^0
  Gain2 : Gain  Gain=2  ParameterDataType=sfix(16)  ParameterScaling=2^0  OutDataType=sfix(16)  OutScaling=2^0
  Gain3 : Gain  Gain=3  ParameterDataType=sfix(16)  ParameterScaling=2^0  OutDataType=sfix(16)  OutScaling=2^0
  Gain4 : Gain  Gain=4  ParameterDataType=sfix(16)  ParameterScaling=2^0  OutDataType=sfix(16)  OutScaling=2^0
  Gain5 : Gain  Gain=5  ParameterDataType=sfix(16)  ParameterScaling=2^0  OutDataType=sfix(16)  OutScaling=2^0
  Gain6 : Gain  Gain=6  ParameterDataType=sfix(16)  ParameterScaling=2^0  OutDataType=sfix(16)  OutScaling=2^0
  MinMax : MinMax  OutDataType=sfix(16)  OutScaling=2^0
  Mux : Mux  Inputs=6
  Sum : Sum  Inputs=-+|  OutDataType=sfix(16)  OutScaling=2^0
  Sum1 : Sum  Inputs=|+-  OutDataType=sfix(16)  OutScaling=2^0
  motohawk_calibration : MotoHawk_lib/Calibration & Probing Blocks/motohawk_calibration  nam='Diff_Ratio'  val=0  storage=Calibration  show_more=on  name_source=Use Parameter  data_type=Inherit from 'Default Value'  read_level=1  write_level=1  ovr_cals=on  view_as=Number  enum_struct={'Disabled', 'Enabled'}  vector_style=Wide Row  use_help_units=off  help=''  units=''  use_header_enum=off  row_header_enum={}  col_header_enum={}  use_min_max=on  min_val=0  max_val=50  use_precision=on  precision='2.3'  gain=1  offset=0  exp=1  use_mototune_group=off  mototune_group=motohawk_vardec_path(gcb)
  motohawk_calibration1 : MotoHawk_lib/Calibration & Probing Blocks/motohawk_calibration  nam='Gear_Ratio_1'  val=0  storage=Calibration  show_more=on  name_source=Use Parameter  data_type=Inherit from 'Default Value'  read_level=1  write_level=1  ovr_cals=on  view_as=Number  enum_struct={'Disabled', 'Enabled'}  vector_style=Wide Row  use_help_units=off  help=''  units=''  use_header_enum=off  row_header_enum={}  col_header_enum={}  use_min_max=on  min_val=0  max_val=50  use_precision=on  precision='1.3'  gain=1  offset=0  exp=1  use_mototune_group=off  mototune_group=motohawk_vardec_path(gcb)
  motohawk_calibration2 : MotoHawk_lib/Calibration & Probing Blocks/motohawk_calibration  nam='Gear_Ratio_2'  val=0  storage=Calibration  show_more=on  name_source=Use Parameter  data_type=Inherit from 'Default Value'  read_level=1  write_level=1  ovr_cals=on  view_as=Number  enum_struct={'Disabled', 'Enabled'}  vector_style=Wide Row  use_help_units=off  help=''  units=''  use_header_enum=off  row_header_enum={}  col_header_enum={}  use_min_max=on  min_val=0  max_val=50  use_precision=on  precision='1.3'  gain=1  offset=0  exp=1  use_mototune_group=off  mototune_group=motohawk_vardec_path(gcb)
  motohawk_calibration3 : MotoHawk_lib/Calibration & Probing Blocks/motohawk_calibration  nam='Gear_Ratio_3'  val=0  storage=Calibration  show_more=on  name_source=Use Parameter  data_type=Inherit from 'Default Value'  read_level=1  write_level=1  ovr_cals=on  view_as=Number  enum_struct={'Disabled', 'Enabled'}  vector_style=Wide Row  use_help_units=off  help=''  units=''  use_header_enum=off  row_header_enum={}  col_header_enum={}  use_min_max=on  min_val=0  max_val=50  use_precision=on  precision='1.3'  gain=1  offset=0  exp=1  use_mototune_group=off  mototune_group=motohawk_vardec_path(gcb)
  motohawk_calibration4 : MotoHawk_lib/Calibration & Probing Blocks/motohawk_calibration  nam='Gear_Ratio_4'  val=0  storage=Calibration  show_more=on  name_source=Use Parameter  data_type=Inherit from 'Default Value'  read_level=1  write_level=1  ovr_cals=on  view_as=Number  enum_struct={'Disabled', 'Enabled'}  vector_style=Wide Row  use_help_units=off  help=''  units=''  use_header_enum=off  row_header_enum={}  col_header_enum={}  use_min_max=on  min_val=0  max_val=50  use_precision=on  precision='1.3'  gain=1  offset=0  exp=1  use_mototune_group=off  mototune_group=motohawk_vardec_path(gcb)
  motohawk_calibration5 : MotoHawk_lib/Calibration & Probing Blocks/motohawk_calibration  nam='Gear_Ratio_5'  val=0  storage=Calibration  show_more=on  name_source=Use Parameter  data_type=Inherit from 'Default Value'  read_level=1  write_level=1  ovr_cals=on  view_as=Number  enum_struct={'Disabled', 'Enabled'}  vector_style=Wide Row  use_help_units=off  help=''  units=''  use_header_enum=off  row_header_enum={}  col_header_enum={}  use_min_max=on  min_val=0  max_val=50  use_precision=on  precision='1.3'  gain=1  offset=0  exp=1  use_mototune_group=off  mototune_group=motohawk_vardec_path(gcb)
  motohawk_calibration6 : MotoHawk_lib/Calibration & Probing Blocks/motohawk_calibration  nam='Gear_Ratio_6'  val=0  storage=Calibration  show_more=on  name_source=Use Parameter  data_type=Inherit from 'Default Value'  read_level=1  write_level=1  ovr_cals=on  view_as=Number  enum_struct={'Disabled', 'Enabled'}  vector_style=Wide Row  use_help_units=off  help=''  units=''  use_header_enum=off  row_header_enum={}  col_header_enum={}  use_min_max=on  min_val=0  max_val=50  use_precision=on  precision='1.3'  gain=1  offset=0  exp=1  use_mototune_group=off  mototune_group=motohawk_vardec_path(gcb)
  gear : Outport  OutDataType=sfix(16)  OutScaling=2^0
  wires:
  In1/1 -> Bus Selector1/1
  Bus Selector1/1 -> Add/1  "<FL_Whl_Spd>"
  Bus Selector1/2 -> Add/2  "<FR_Whl_Spd>"
  Add/1 -> Gain/1
  Gain/1 -> Divide/1
  motohawk_calibration/1 -> Divide/2
  Divide1/1 -> Sum/2
  Bus Selector1/3 -> Sum/1  "<Eng_Spd>"
  motohawk_calibration1/1 -> Mux/1
  motohawk_calibration2/1 -> Mux/2
  motohawk_calibration3/1 -> Mux/3
  motohawk_calibration4/1 -> Mux/4
  motohawk_calibration5/1 -> Mux/5
  motohawk_calibration6/1 -> Mux/6
  Mux/1 -> Divide1/2
  Divide/1 -> Divide1/1
  Sum/1 -> Abs/1
  MinMax/1 -> Sum1/2
  Abs/1 -> Sum1/1, MinMax/1
  Sum1/1 -> Compare To Zero1/1
  Compare To Zero1/1 -> Demux/1
  Demux/1 -> Gain1/1
  Demux/2 -> Gain2/1
  Demux/3 -> Gain3/1
  Demux/4 -> Gain4/1
  Demux/5 -> Gain5/1
  Demux/6 -> Gain6/1
  Gain1/1 -> Add1/1
  Gain2/1 -> Add1/2
  Gain3/1 -> Add1/3
  Gain4/1 -> Add1/4
  Gain5/1 -> Add1/5
  Gain6/1 -> Add1/6
  Add1/1 -> gear/1

== system cx06_MA/Strategy/Fiat/GMLAN Control Code/Neutral Check ==
  gear_In : Inport  OutDataType=sfix(16)  OutScaling=2^0
  In1 : Inport  Port=2  OutDataType=sfix(16)  OutScaling=2^0
  Bus Selector : BusSelector  OutputSignals=Analog.Trans.Reverse,Analog.Trans.Neutral
  Compare To Zero : simulink/Logic and Bit Operations/Compare To Zero  SystemSampleTime=-1  relop=~=  LogicOutDataTypeMode=boolean  ZeroCross=off
  Logical Operator : Logic  Operator=OR  AllPortsSameDT=off  OutDataTypeMode=boolean  OutDataTypeStr=boolean
  Logical Operator1 : Logic  AllPortsSameDT=off  OutDataTypeMode=boolean  OutDataTypeStr=boolean
  fault : Outport  OutDataType=sfix(16)  OutScaling=2^0
  wires:
  In1/1 -> Bus Selector/1
  gear_In/1 -> Compare To Zero/1
  Compare To Zero/1 -> Logical Operator/1
  Bus Selector/1 -> Logical Operator/2  "<Reverse>"
  Logical Operator/1 -> Logical Operator1/1
  Bus Selector/2 -> Logical Operator1/2  "<Neutral>"
  Logical Operator1/1 -> fault/1

== system cx06_MA/Strategy/Hybrid Control Code/Activation of Accel Through Shifts ==
  Inputs : Inport  OutDataType=sfix(16)  OutScaling=2^0
  Bus Selector : BusSelector  OutputSignals=Analog.Driver.Clutch,GMLAN.Park_Brake,Analog.Driver.Brake,Analog.Driver.Accel,Analog.Trans.Neutral,IPT.Status 2.veh_speed
  Engine_Running : Stateflow chart  TreatAsAtomicUnit=on
  Logical Operator : Logic  AllPortsSameDT=off  OutDataTypeMode=boolean  OutDataTypeStr=boolean
  Relational Operator : RelationalOperator  Operator=>  LogicOutDataTypeMode=boolean  OutDataTypeStr=boolean
  Relational Operator1 : RelationalOperator  Operator=<  LogicOutDataTypeMode=Specify via dialog  OutDataTypeStr=uint(8)
  Relational Operator2 : RelationalOperator  Operator=<  LogicOutDataTypeMode=Specify via dialog  OutDataTypeStr=uint(8)
  Relational Operator3 : RelationalOperator  Operator=<  LogicOutDataTypeMode=Specify via dialog  OutDataTypeStr=uint(8)
  motohawk_calibration1 : MotoHawk_lib/Calibration & Probing Blocks/motohawk_calibration  nam='EnableSport'  val=1  storage=Calibration  show_more=on  name_source=Use Parameter  data_type=uint8  read_level=1  write_level=1  ovr_cals=on  view_as=Enumeration  enum_struct={'False', 'True'}  vector_style=Wide Row  use_help_units=off  help=''  units=''  use_header_enum=off  row_header_enum={}  col_header_enum={}  use_min_max=off  min_val=-inf  max_val=inf  use_precision=off  precision=''  gain=1  offset=0  exp=1  use_mototune_group=off  mototune_group=motohawk_vardec_path(gcb)
  motohawk_calibration2 : MotoHawk_lib/Calibration & Probing Blocks/motohawk_calibration  nam='Activation_Spd'  val=5  storage=Calibration  show_more=on  name_source=Use Parameter  data_type=double  read_level=1  write_level=1  ovr_cals=on  view_as=Number  enum_struct={'False', 'True'}  vector_style=Wide Row  use_help_units=off  help=''  units=''  use_header_enum=off  row_header_enum={}  col_header_enum={}  use_min_max=on  min_val=0  max_val=inf  use_precision=off  precision=''  gain=1  offset=0  exp=1  use_mototune_group=off  mototune_group=motohawk_vardec_path(gcb)
  motohawk_calibration3 : MotoHawk_lib/Calibration & Probing Blocks/motohawk_calibration  nam='Accel_Pedal_Pos'  val=.5  storage=Calibration  show_more=on  name_source=Use Parameter  data_type=double  read_level=1  write_level=1  ovr_cals=on  view_as=Number  enum_struct={'False', 'True'}  vector_style=Wide Row  use_help_units=off  help=''  units=''  use_header_enum=off  row_header_enum={}  col_header_enum={}  use_min_max=on  min_val=0  max_val=1  use_precision=on  precision='1.2'  gain=1  offset=0  exp=1  use_mototune_group=off  mototune_group=motohawk_vardec_path(gcb)
  motohawk_calibration9 : MotoHawk_lib/Calibration & Probing Blocks/motohawk_calibration  nam='Clutch_Mech_Engage_in_Accel_Through_Shifts'  val=0.75  storage=Calibration  show_more=off  name_source=Use Parameter  data_type=Inherit from 'Default Value'  read_level=1  write_level=1  ovr_cals=on  view_as=Number  enum_struct={'Disabled', 'Enabled'}  vector_style=Wide Row  use_help_units=off  help=''  units=''  use_header_enum=off  row_header_enum={}  col_header_enum={}  use_min_max=off  min_val=-inf  max_val=inf  use_precision=off  precision=''  gain=1  offset=0  exp=1  use_mototune_group=off  mototune_group=motohawk_vardec_path(gcb)
  motohawk_data_read1 : MotoHawk_lib/Data Storage Blocks/motohawk_data_read  source=Lookup By Name  structure=Scalar  operation=Read scalar from location by index  sz_vec=4  sz_row=2  sz_col=3  typ=double  nam='Regen_Start'  checkNull=on  struct_inst_name='Struct1'  struct_nam='MyStruct'
  motohawk_probe2 : MotoHawk_lib/Calibration & Probing Blocks/motohawk_probe  nam='Sport_Mode'  show_more=on  name_source=Use Parameter  read_level=1  view_as=Number  enum_struct={'Disabled', 'Enabled'}  vector_style=Wide Row  use_help_units=off  help=''  units=''  use_header_enum=off  row_header_enum={}  col_header_enum={}  use_precision=off  precision=''  gain=1  offset=0  exp=1  use_mototune_group=off  mototune_group=motohawk_vardec_path(gcb)
  Sport_Mode : Outport  OutDataType=sfix(16)  OutScaling=2^0
  wires:
  Inputs/1 -> Bus Selector/1
  Bus Selector/6 -> Relational Operator/1  "<veh_speed>"
  motohawk_calibration2/1 -> Relational Operator/2
  Logical Operator/1 -> Sport_Mode/1, motohawk_probe2/1
  motohawk_calibration1/1 -> Logical Operator/2
  Engine_Running/1(output) -> Logical Operator/1
  motohawk_calibration9/1 -> Relational Operator1/1
  Bus Selector/1 -> Relational Operator1/2  "<Clutch>"
  Relational Operator1/1 -> Engine_Running/1(Clutching)
  Bus Selector/2 -> Engine_Running/2(EBrake)  "<Park_Brake>"
  Bus Selector/3 -> Relational Operator2/2  "<Brake>"
  Relational Operator/1 -> Engine_Running/6(spd)
  Bus Selector/5 -> Engine_Running/5(Neutral)  "<Neutral>"
  motohawk_data_read1/1 -> Relational Operator2/1
  Relational Operator2/1 -> Engine_Running/3(Braking)
  Bus Selector/4 -> Relational Operator3/2  "<Accel>"
  motohawk_calibration3/1 -> Relational Operator3/1
  Relational Operator3/1 -> Engine_Running/4(Acceling)

== system cx06_MA/Strategy/Hybrid Control Code/Activation of Assisted Take-off ==
  In1 : Inport  OutDataType=sfix(16)  OutScaling=2^0
  Bus Selector3 : BusSelector  OutputSignals=Analog.Driver.Clutch,IPT.Status 2.veh_speed
  Chart : Stateflow chart  TreatAsAtomicUnit=on
  motohawk_calibration4 : MotoHawk_lib/Calibration & Probing Blocks/motohawk_calibration  nam='AT_Enable'  val=1  storage=Calibration  show_more=on  name_source=Use Parameter  data_type=uint8  read_level=1  write_level=1  ovr_cals=on  view_as=Enumeration  enum_struct={'Disabled', 'Enabled'}  vector_style=Wide Row  use_help_units=on  help='Enables Assisted Takeoff'  units=''  use_header_enum=off  row_header_enum={}  col_header_enum={}  use_min_max=off  min_val=0  max_val=1  use_precision=on  precision=''  gain=1  offset=0  exp=1  use_mototune_group=off  mototune_group=motohawk_vardec_path(gcb)
  motohawk_data_read : MotoHawk_lib/Data Storage Blocks/motohawk_data_read  source=Lookup By Name  structure=Scalar  operation=Read scalar from location by index  sz_vec=4  sz_row=2  sz_col=3  typ=double  nam='AT_Start'  checkNull=on  struct_inst_name='Struct1'  struct_nam='MyStruct'
  motohawk_data_read1 : MotoHawk_lib/Data Storage Blocks/motohawk_data_read  source=Lookup By Name  structure=Scalar  operation=Read scalar from location by index  sz_vec=4  sz_row=2  sz_col=3  typ=double  nam='AT_Stop'  checkNull=on  struct_inst_name='Struct1'  struct_nam='MyStruct'
  motohawk_probe : MotoHawk_lib/Calibration & Probing Blocks/motohawk_probe  nam='AT_Active'  show_more=on  name_source=Use Parameter  read_level=1  view_as=Enumeration  enum_struct={'False', 'True'}  vector_style=Wide Row  use_help_units=off  help=''  units=''  use_header_enum=off  row_header_enum={}  col_header_enum={}  use_precision=off  precision=''  gain=1  offset=0  exp=1  use_mototune_group=off  mototune_group=motohawk_vardec_path(gcb)
  Active? : Outport  OutDataType=sfix(16)  OutScaling=2^0
  wires:
  motohawk_data_read/1 -> Chart/1(Start)
  motohawk_data_read1/1 -> Chart/2(Stop)
  Bus Selector3/1 -> Chart/3(clutch)  "<Clutch>"
  Bus Selector3/2 -> Chart/4(speed)  "<veh_speed>"
  motohawk_calibration4/1 -> Chart/5(enabled)
  In1/1 -> Bus Selector3/1
  Chart/1(active) -> Active?/1, motohawk_probe/1
